simulink model "lab_1_n_3"  (R2021b)
settings: Solver=VariableStepAuto  StartTime=0.0  StopTime=100.0  RelTol=1e-3
settings Model: Creator=peter  LastModifiedBy=peter

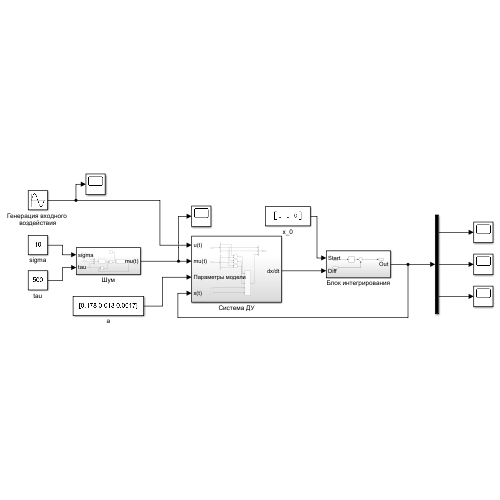
[thumbnail: Simulink's stored preview of the top-level diagram]
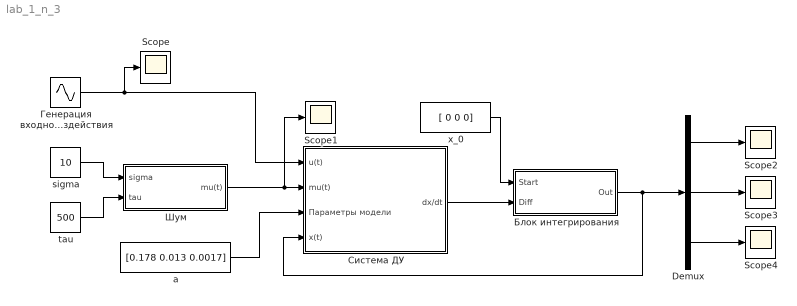
== system lab_1_n_3 ==
  Demux : Demux  Outputs=3
  Scope{,1..4} (5 alike) : Scope
  a : Constant  Value=[0.178 0.013 0.0017]
  sigma : Constant  Value=10
  tau : Constant  Value=500
  x_0 : Constant  Value=[ 0 0 0]
  Блок интегрирования : Subsystem
  Генерация входного воздействия : Sin  Frequency=0.05  SampleTime=0
  Система ДУ : Subsystem
  Шум : Subsystem
  wires:
  Demux/1 -> Scope2/1
  Demux/2 -> Scope3/1
  Demux/3 -> Scope4/1
  Блок интегрирования/1(Out) -> Система ДУ/4(x(t)), Demux/1
  x_0/1 -> Блок интегрирования/1(Start)
  Система ДУ/1(dx/dt) -> Блок интегрирования/2(Diff)
  a/1 -> Система ДУ/3(Параметры модели)
  Шум/1(mu(t)) -> Scope1/1, Система ДУ/2(mu(t))
  tau/1 -> Шум/2(tau)
  sigma/1 -> Шум/1(sigma)
  Генерация входного воздействия/1 -> Scope/1, Система ДУ/1(u(t))

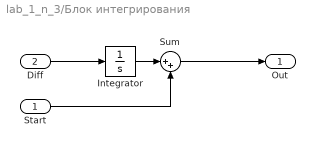
== system lab_1_n_3/Блок интегрирования ==
  Start : Inport
  Diff : Inport  Port=2
  Integrator : Integrator
  Sum : Sum  Inputs=|++
  Out : Outport
  wires:
  Diff/1 -> Integrator/1
  Sum/1 -> Out/1
  Integrator/1 -> Sum/1
  Start/1 -> Sum/2

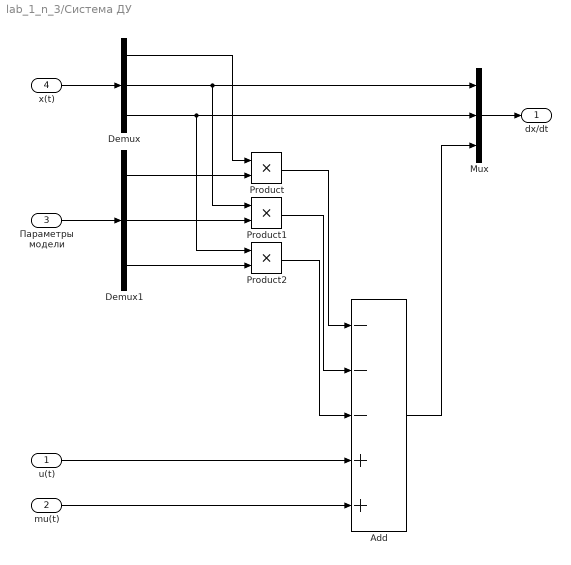
== system lab_1_n_3/Система ДУ ==
  u(t) : Inport
  mu(t) : Inport  Port=2
  Параметры модели : Inport  Port=3
  x(t) : Inport  Port=4
  Add : Sum  Inputs=---++
  Demux : Demux  Outputs=3
  Demux1 : Demux  Outputs=3
  Mux : Mux  Inputs=3
  Product : Product
  Product1 : Product
  Product2 : Product
  dx/dt : Outport
  wires:
  x(t)/1 -> Demux/1
  Параметры модели/1 -> Demux1/1
  Mux/1 -> dx/dt/1
  u(t)/1 -> Add/4
  mu(t)/1 -> Add/5
  Demux1/1 -> Product/2
  Demux1/2 -> Product1/2
  Demux1/3 -> Product2/2
  Demux/1 -> Product/1
  Demux/2 -> Mux/1, Product1/1
  Demux/3 -> Mux/2, Product2/1
  Add/1 -> Mux/3
  Product/1 -> Add/1
  Product1/1 -> Add/2
  Product2/1 -> Add/3

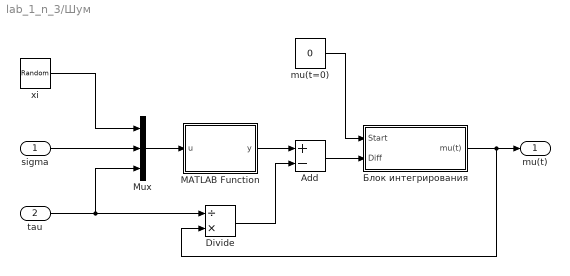
== system lab_1_n_3/Шум ==
  sigma : Inport
  tau : Inport  Port=2
  Add : Sum  Inputs=+-
  Divide : Product  Inputs=/*
  MATLAB Function : MATLAB Function  TreatAsAtomicUnit=on
  Mux : Mux  Inputs=3
  mu(t=0) : Constant  Value=0
  xi : RandomNumber  SampleTime=0.1
  Блок интегрирования : Subsystem
  mu(t) : Outport
  wires:
  mu(t=0)/1 -> Блок интегрирования/1(Start)
  Блок интегрирования/1(mu(t)) -> Divide/2, mu(t)/1
  xi/1 -> Mux/1
  sigma/1 -> Mux/2
  tau/1 -> Divide/1, Mux/3
  Add/1 -> Блок интегрирования/2(Diff)
  Divide/1 -> Add/2
  MATLAB Function/1(y) -> Add/1
  Mux/1 -> MATLAB Function/1(u)

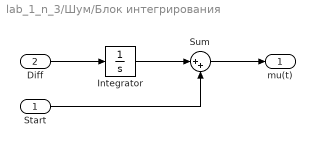
== system lab_1_n_3/Шум/Блок интегрирования ==
  Start : Inport
  Diff : Inport  Port=2
  Integrator : Integrator
  Sum : Sum  Inputs=|++
  mu(t) : Outport
  wires:
  Integrator/1 -> Sum/1
  Sum/1 -> mu(t)/1
  Diff/1 -> Integrator/1
  Start/1 -> Sum/2

== matlab function lab_1_n_3/Шум/MATLAB Function ==
  data: u input; y output
function y = fcn(u)
    xi=u(1);
    sigma=u(2);
    tau=u(3);
    alpha=1/tau;
    k_f=sigma*sqrt(2*alpha);
y = k_f*xi;
